simulink model "Two_prot_mod"  (R2021a)
settings: Solver=VariableStepAuto  StartTime=0.0  StopTime=100  RelTol=1e-3
model workspace (MATLAB code in the model file):
  | Kab=12;
  | Kia=10;
  | kba=8;
  | Fb=2;
  | kfb=1;
  | I=0.3
  | Kba=8;
  | x_star =[Fb/Kba;Kia*(Kba-Fb)*I/(Kab*Fb)];
settings Model: Creator=priya  LastModifiedBy=Priyan_PC
settings SolverCC: AlgebraicLoopSolver=TrustRegion
settings DebuggingCC: SFMachineParentedDataDiag=warning

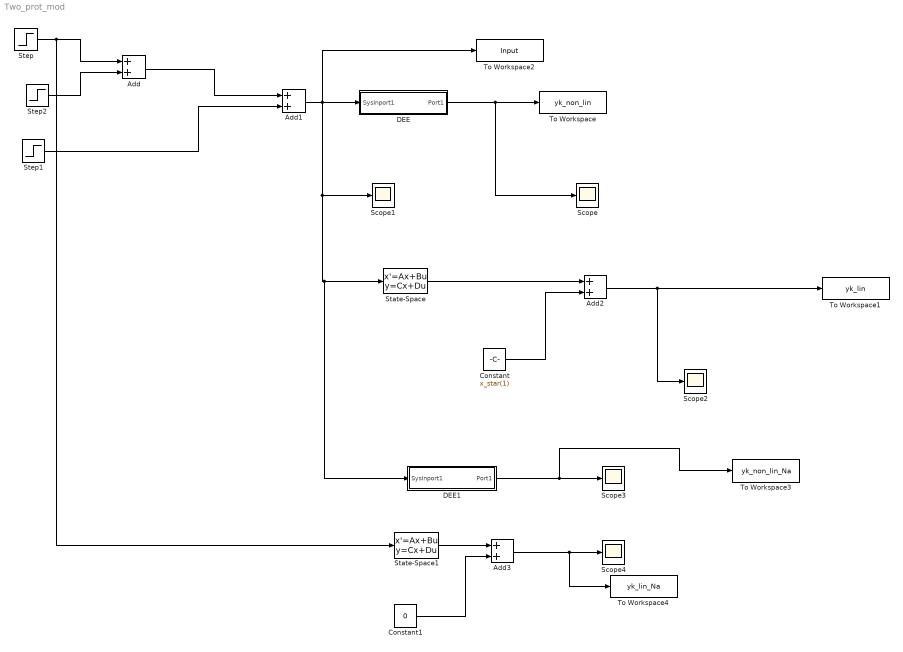
== system Two_prot_mod ==
  Add{,1..3} (4 alike) : Sum
  Constant : Constant  Value=x_star(1)
  Constant1 : Constant  Value=0
  DEE : Subsystem  mask(Differential Equation Editor (DEE)){}
      settings: OpenFcn=diffeqed
      mask Display: disp('Differential Equation\n Editor')
  DEE1 : Subsystem  mask(Differential Equation Editor (DEE)){}
      settings: OpenFcn=diffeqed
      mask Display: disp('Differential Equation\n Editor')
  Scope{,1..4} (5 alike) : Scope
  State-Space : StateSpace  A=[-9 -3;8 0]  B=[7.5;0]  C=[1 0]  D=0  InitialCondition=0
  State-Space1 : StateSpace  A=[-1 -0.15*1.8; 1 0]  B=[1;0]  C=[1 0]  D=0  InitialCondition=0
  Step : Step  Time=0  Before=0.3  After=0.5  SampleTime=0
  Step1 : Step  Time=10  After=-0.2  SampleTime=0
  Step2 : Step  Time=18  After=0.2  SampleTime=0
  To Workspace : ToWorkspace  VariableName=yk_non_lin  SampleTime=-1
  To Workspace1 : ToWorkspace  VariableName=yk_lin  SampleTime=-1
  To Workspace2 : ToWorkspace  VariableName=Input  SampleTime=-1
  To Workspace3 : ToWorkspace  VariableName=yk_non_lin_Na  SampleTime=-1
  To Workspace4 : ToWorkspace  VariableName=yk_lin_Na  SampleTime=-1
  wires:
  DEE/1(Port1) -> Scope/1, To Workspace/1
  Step/1 -> State-Space1/1, Add/1
  Step2/1 -> Add/2
  Add/1 -> Add1/1
  Step1/1 -> Add1/2
  Add1/1 -> To Workspace2/1, DEE1/1(SysInport1), State-Space/1, Scope1/1, DEE/1(SysInport1)
  State-Space/1 -> Add2/1
  Constant/1 -> Add2/2
  Add2/1 -> Scope2/1, To Workspace1/1
  DEE1/1(Port1) -> To Workspace3/1, Scope3/1
  Constant1/1 -> Add3/2
  State-Space1/1 -> Add3/1
  Add3/1 -> To Workspace4/1, Scope4/1

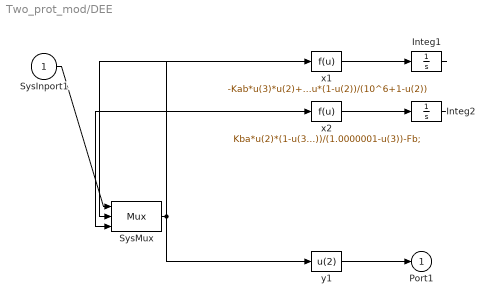
== system Two_prot_mod/DEE ==
  SysInport1 : Inport
  Integ1 : Integrator  InitialCondition=x_star(1)
  Integ2 : Integrator  InitialCondition=x_star(2)
  SysMux : Mux  Inputs=3
  x1 : Fcn  Expr=-Kab*u(3)*u(2)+10^7*u*(1-u(2))/(10^6+1-u(2))
  x2 : Fcn  Expr=Kba*u(2)*(1-u(3))/(1.0000001-u(3))-Fb;
  y1 : Fcn  Expr=u(2)
  Port1 : Outport
  wires:
  SysInport1/1 -> SysMux/1
  SysMux/1 -> x1/1, x2/1, y1/1
  x1/1 -> Integ1/1
  Integ1/1 -> SysMux/2
  x2/1 -> Integ2/1
  Integ2/1 -> SysMux/3
  y1/1 -> Port1/1

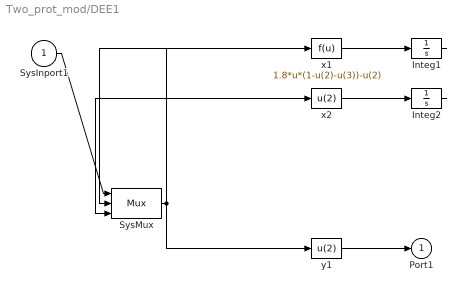
== system Two_prot_mod/DEE1 ==
  SysInport1 : Inport
  Integ1 : Integrator  InitialCondition=0;
  Integ2 : Integrator
  SysMux : Mux  Inputs=3
  x1 : Fcn  Expr=1.8*u*(1-u(2)-u(3))-u(2)
  x2 : Fcn  Expr=u(2)
  y1 : Fcn  Expr=u(2)
  Port1 : Outport
  wires:
  SysInport1/1 -> SysMux/1
  SysMux/1 -> x1/1, x2/1, y1/1
  x1/1 -> Integ1/1
  Integ1/1 -> SysMux/2
  x2/1 -> Integ2/1
  Integ2/1 -> SysMux/3
  y1/1 -> Port1/1
